simulink model "transfer"  (R2013b)
settings: Solver=ode45  StartTime=0.0  StopTime=10.0  RelTol=1e-3
values from neighbouring files (symbols this model uses):
  a = 0.001    [transfer.m]
  J = 0.00025    [transfer.m]
  K = 0.05    [transfer.m]
  R = 0.5    [transfer.m]
settings Model: Creator=daniw  LastModifiedBy=daniw

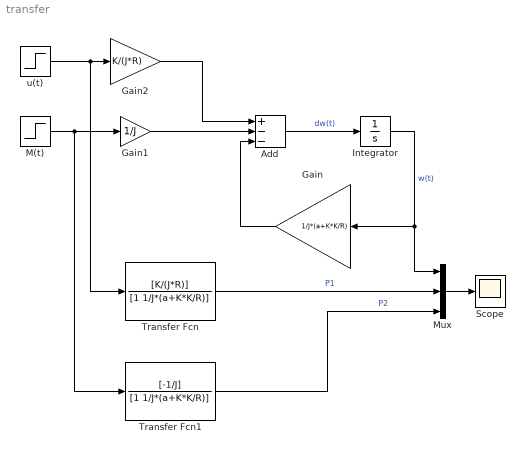
== system transfer ==
  Add : Sum  Inputs=+--
  Gain : Gain  Gain=1/J*(a+K*K/R)
  Gain1 : Gain  Gain=1/J
  Gain2 : Gain  Gain=K/(J*R)
  Integrator : Integrator
  M(t) : Step  Time=2  SampleTime=0
  Mux : Mux  Inputs=3
  Scope : Scope
  Transfer Fcn : TransferFcn  Numerator=[K/(J*R)]  Denominator=[1 1/J*(a+K*K/R)]
  Transfer Fcn1 : TransferFcn  Numerator=[-1/J]  Denominator=[1 1/J*(a+K*K/R)]
  u(t) : Step  Before=5  After=20  SampleTime=0
  wires:
  Add/1 -> Integrator/1  "dw(t)"
  Integrator/1 -> Mux/1, Gain/1  "w(t)"
  Gain/1 -> Add/3
  M(t)/1 -> Transfer Fcn1/1, Gain1/1
  Gain1/1 -> Add/2
  u(t)/1 -> Transfer Fcn/1, Gain2/1
  Gain2/1 -> Add/1
  Mux/1 -> Scope/1
  Transfer Fcn/1 -> Mux/2  "P1"
  Transfer Fcn1/1 -> Mux/3  "P2"
